simulink library "Spring_AirOilPiston"  (R2026a)
settings: Solver=VariableStepAuto
undefined symbols (not defined in the file): Spring
libraries: fl_lib x46, nesl_utility x25, SimscapeFluids_lib x13, sdl_lib x2
(part 4 of 6)

== system Spring_AirOilPiston/AirOilPiston/Sensor Gas Stiff T  ==
  PS-Simulink Converter10 : nesl_utility/PS-Simulink Converter  PhysicalDomain=network_engine_domain  SubClassName=ps_output  LeftPortType=input  RightPortType=output  PseudoPeriodic=off  Frequencies=[]  VectorFormat=inherit  Unit=degC  AffineConversion=on
  Temperature Sensor : fl_lib/Thermal/Thermal Sensors/Temperature Sensor  temperature_measure=foundation.enum.MeasurementReference.difference
  ThRef : fl_lib/Thermal/Thermal Elements/Thermal Reference
  A : PMIOPort  Side=Left
  T : Outport
  wires:
  PS-Simulink Converter10/1 -> T/1
  connections:
  A/RConn1 -- Temperature Sensor/LConn1
  PS-Simulink Converter10/LConn1 -- Temperature Sensor/RConn2
  ThRef/LConn1 -- Temperature Sensor/RConn1
